simulink model "P4_Like"  (R2015b)
settings: Solver=VariableStepAuto  StartTime=0.0  StopTime=100  RelTol=1e-3
values from neighbouring files (symbols this model uses):
  B = 0.1    [Parameters.m]    (also in controller2.m = b/tsampling * eye(3,3))
  Dm = 0.2    [Parameters.m]
  Ds = 0.1    [Parameters.m]
  K = ceil(max(K1,K2))    [Gains.m]
  Lm1 = 0.5    [Parameters.m]
  Lm2 = 0.5    [Parameters.m]
  Ls1 = 0.5    [Parameters.m]
  Ls2 = 0.5    [Parameters.m]
  Mm1 = 1    [Parameters.m]
  Mm2 = 1    [Parameters.m]
  Ms1 = 2    [Parameters.m]
  Ms2 = 2    [Parameters.m]
  P = 10    [Parameters.m]
  q0 = [0;0]    [Parameters.m]
  v0 = [0;0;0]    [Initiation.m]    (also in Parameters.m = [0;0])
settings Model: Creator=TOSHIBA  LastModifiedBy=TOSHIBA

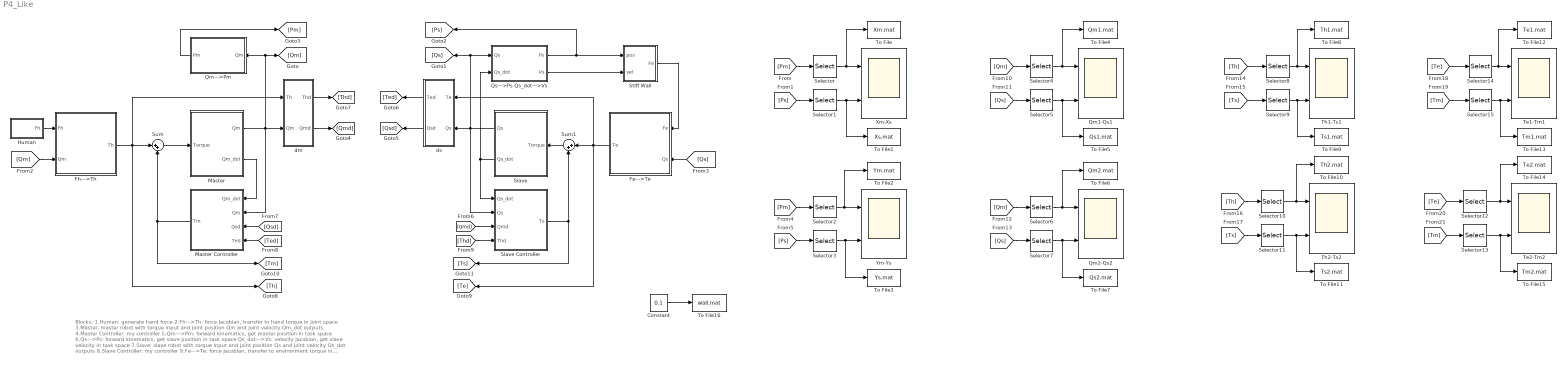
== system P4_Like ==
  note: Blocks:
      | 1.Human: generate hand force
      | 2.Fh--->Th: force Jacobian, transfer to hand torque in joint space
      | 3.Master: master robot with torque input and joint position Qm and joint velocity Qm_dot outputs
      | 4.Master Controller: my controller
      | 5.Qm--->Pm: forward kinematics, get master position in task space
      | 6.Qs--->Ps: forward kinematics, get slave position in task space
      | Qs_dot--->Vs: velocity jacobian, get slave velocity in task space
      | 7.Slave: slave robot with torque input and joint position Qs and joint velocity Qs_dot outputs
      | 8.Slave Controller: my controller
      | 9.Fe--->Te: force Jacobian, transfer to environment torque in joint space
      | 10.Stiff Wall: spring with k=10KN/m, active damping d=40Ns/m
  Constant : Constant  Value=0.1
  Fe--->Te : Subsystem
  Fh--->Th : Subsystem
  Human : Subsystem
  Master : Subsystem
  Master Controller : Subsystem
  Qm--->Pm : Subsystem
  Qm1-Qs1 : Scope  NumInputPorts=2
  Qm2-Qs2 : Scope  NumInputPorts=2
  Qs--->Ps Qs_dot--->Vs : Subsystem
  Selector{,1,4..5,8..9,14..15} (8 alike) : Selector  InputPortWidth=2  IndexOptions=Index vector (dialog)  Indices=[1]  OutputSizes=1
  Selector{2..3,6..7,10..13} (8 alike) : Selector  InputPortWidth=2  IndexOptions=Index vector (dialog)  Indices=[2]  OutputSizes=1
  Slave : Subsystem
  Slave Controller : Subsystem
  Stiff Wall : Subsystem
  Sum : Sum  Inputs=|++
  Sum1 : Sum  Inputs=|++
  Te1-Tm1 : Scope  NumInputPorts=2
  Te2-Tm2 : Scope  NumInputPorts=2
  Th1-Ts1 : Scope  NumInputPorts=2
  Th2-Ts2 : Scope  NumInputPorts=2
  To File : ToFile  Filename=Xm.mat  MatrixName=Xm  SaveFormat=Timeseries
  To File1 : ToFile  Filename=Xs.mat  MatrixName=Xs  SaveFormat=Timeseries
  To File10 : ToFile  Filename=Th2.mat  MatrixName=Th2  SaveFormat=Timeseries
  To File11 : ToFile  Filename=Ts2.mat  MatrixName=Ts2  SaveFormat=Timeseries
  To File12 : ToFile  Filename=Te1.mat  MatrixName=Te1  SaveFormat=Timeseries
  To File13 : ToFile  Filename=Tm1.mat  MatrixName=Tm1  SaveFormat=Timeseries
  To File14 : ToFile  Filename=Te2.mat  MatrixName=Te2  SaveFormat=Timeseries
  To File15 : ToFile  Filename=Tm2.mat  MatrixName=Tm2  SaveFormat=Timeseries
  To File16 : ToFile  Filename=wall.mat  MatrixName=wall  SaveFormat=Timeseries
  To File2 : ToFile  Filename=Ym.mat  MatrixName=Ym  SaveFormat=Timeseries
  To File3 : ToFile  Filename=Ys.mat  MatrixName=Ys  SaveFormat=Timeseries
  To File4 : ToFile  Filename=Qm1.mat  MatrixName=Qm1  SaveFormat=Timeseries
  To File5 : ToFile  Filename=Qs1.mat  MatrixName=Qs1  SaveFormat=Timeseries
  To File6 : ToFile  Filename=Qm2.mat  MatrixName=Qm2  SaveFormat=Timeseries
  To File7 : ToFile  Filename=Qs2.mat  MatrixName=Qs2  SaveFormat=Timeseries
  To File8 : ToFile  Filename=Th1.mat  MatrixName=Th1  SaveFormat=Timeseries
  To File9 : ToFile  Filename=Ts1.mat  MatrixName=Ts1  SaveFormat=Timeseries
  Xm-Xs : Scope  NumInputPorts=2
  Ym-Ys : Scope  NumInputPorts=2
  dm : Subsystem
  ds : Subsystem
  wires:
  Qs--->Ps Qs_dot--->Vs/1(Ps) -> Stiff Wall/1(pos), [Ps]
  Fe--->Te/1(Te) -> [Te], ds/1(Te), Sum1/1
  Sum1/1 -> Slave/1(Torque)
  Sum/1 -> Master/1(Torque)
  Fh--->Th/1(Th) -> [Th], dm/1(Th), Sum/1
  Master/2(Qm_dot) -> Master Controller/1(Qm_dot)
  Master Controller/1(Tm) -> [Tm], Sum/2
  Slave/2(Qs_dot) -> Qs--->Ps Qs_dot--->Vs/2(Qs_dot), Slave Controller/1(Qs_dot)
  Slave Controller/1(Ts) -> [Ts], Sum1/2
  [Qs] -> Fe--->Te/2(Qs)
  Master/1(Qm) -> Master Controller/2(Qm), dm/2(Qm), [Qm], Qm--->Pm/1(Qm)
  Slave/1(Qs) -> ds/2(Qs), [Qs], Qs--->Ps Qs_dot--->Vs/1(Qs), Slave Controller/2(Qs)
  [Qm] -> Fh--->Th/2(Qm)
  Human/1(Fh) -> Fh--->Th/1(Fh)
  Qm--->Pm/1(Pm) -> [Pm]
  [Pm] -> Selector/1
  Selector/1 -> To File/1, Xm-Xs/1
  [Ps] -> Selector1/1
  Selector1/1 -> To File1/1, Xm-Xs/2
  [Pm] -> Selector2/1
  Selector2/1 -> To File2/1, Ym-Ys/1
  [Ps] -> Selector3/1
  Selector3/1 -> To File3/1, Ym-Ys/2
  [Qmd] -> Slave Controller/3(Qmd)
  [Qsd] -> Master Controller/3(Qsd)
  [Ted] -> Master Controller/4(Ted)
  ds/2(Qsd) -> [Qsd]
  ds/1(Ted) -> [Ted]
  dm/2(Qmd) -> [Qmd]
  dm/1(Thd) -> [Thd]
  [Thd] -> Slave Controller/4(Thd)
  [Qs] -> Selector5/1
  [Qm] -> Selector4/1
  Selector4/1 -> To File4/1, Qm1-Qs1/1
  Selector5/1 -> To File5/1, Qm1-Qs1/2
  [Qs] -> Selector7/1
  [Qm] -> Selector6/1
  Selector6/1 -> To File6/1, Qm2-Qs2/1
  Selector7/1 -> To File7/1, Qm2-Qs2/2
  [Th] -> Selector8/1
  [Ts] -> Selector9/1
  Selector9/1 -> To File9/1, Th1-Ts1/2
  Selector8/1 -> To File8/1, Th1-Ts1/1
  [Ts] -> Selector11/1
  [Th] -> Selector10/1
  Selector10/1 -> To File10/1, Th2-Ts2/1
  [Te] -> Selector14/1
  [Tm] -> Selector15/1
  Selector15/1 -> To File13/1, Te1-Tm1/2
  Selector14/1 -> To File12/1, Te1-Tm1/1
  [Tm] -> Selector13/1
  [Te] -> Selector12/1
  Selector12/1 -> To File14/1, Te2-Tm2/1
  Selector13/1 -> To File15/1, Te2-Tm2/2
  Selector11/1 -> To File11/1, Th2-Ts2/2
  Constant/1 -> To File16/1
  Qs--->Ps Qs_dot--->Vs/2(Vs) -> Stiff Wall/2(vel)
  Stiff Wall/1(Fe) -> Fe--->Te/1(Fe)

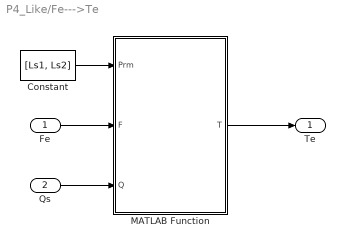
== system P4_Like/Fe--->Te ==
  Fe : Inport
  Qs : Inport  Port=2
  Constant : Constant  Value=[Ls1, Ls2]
  MATLAB Function : MATLAB Function  TreatAsAtomicUnit=on
  Te : Outport
  wires:
  Qs/1 -> MATLAB Function/3(Q)
  Fe/1 -> MATLAB Function/2(F)
  MATLAB Function/1(T) -> Te/1
  Constant/1 -> MATLAB Function/1(Prm)

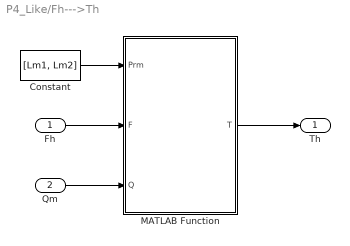
== system P4_Like/Fh--->Th ==
  Fh : Inport
  Qm : Inport  Port=2
  Constant : Constant  Value=[Lm1, Lm2]
  MATLAB Function : MATLAB Function  TreatAsAtomicUnit=on
  Th : Outport
  wires:
  Fh/1 -> MATLAB Function/2(F)
  MATLAB Function/1(T) -> Th/1
  Qm/1 -> MATLAB Function/3(Q)
  Constant/1 -> MATLAB Function/1(Prm)

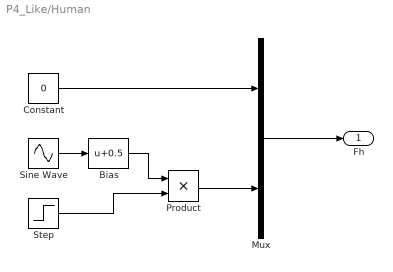
== system P4_Like/Human ==
  Bias : Bias  Bias=0.5
  Constant : Constant  Value=0
  Mux : Mux  Inputs=2
  Product : Product
  Sine Wave : Sin  Frequency=pi/20  SampleTime=0
  Step : Step  Time=100  Before=1  After=0  SampleTime=0
  Fh : Outport
  wires:
  Mux/1 -> Fh/1
  Constant/1 -> Mux/1
  Step/1 -> Product/2
  Bias/1 -> Product/1
  Product/1 -> Mux/2
  Sine Wave/1 -> Bias/1

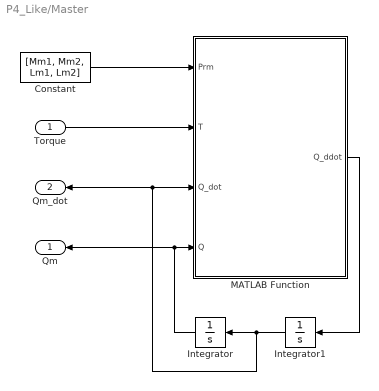
== system P4_Like/Master ==
  Torque : Inport
  Constant : Constant  Value=[Mm1, Mm2, Lm1, Lm2]
  Integrator : Integrator  InitialCondition=q0
  Integrator1 : Integrator  InitialCondition=v0
  MATLAB Function : MATLAB Function  TreatAsAtomicUnit=on
  Qm : Outport
  Qm_dot : Outport  Port=2
  wires:
  Torque/1 -> MATLAB Function/2(T)
  Constant/1 -> MATLAB Function/1(Prm)
  MATLAB Function/1(Q_ddot) -> Integrator1/1
  Integrator1/1 -> MATLAB Function/3(Q_dot), Qm_dot/1, Integrator/1
  Integrator/1 -> MATLAB Function/4(Q), Qm/1

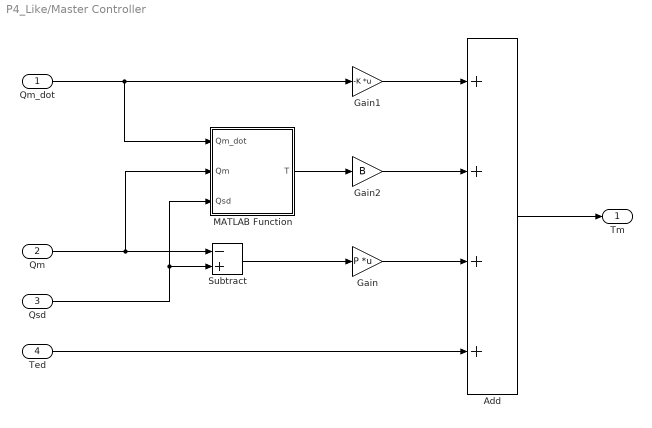
== system P4_Like/Master Controller ==
  Qm_dot : Inport
  Qm : Inport  Port=2
  Qsd : Inport  Port=3
  Ted : Inport  Port=4
  Add : Sum  Inputs=++++
  Gain : Gain  Gain=P  Multiplication=Matrix(K*u) (u vector)
  Gain1 : Gain  Gain=-K  Multiplication=Matrix(K*u) (u vector)
  Gain2 : Gain  Gain=B
  MATLAB Function : MATLAB Function  TreatAsAtomicUnit=on
  Subtract : Sum  Inputs=-+
  Tm : Outport
  wires:
  Qm/1 -> MATLAB Function/2(Qm), Subtract/1
  Qsd/1 -> Subtract/2, MATLAB Function/3(Qsd)
  Gain/1 -> Add/3
  Gain1/1 -> Add/1
  Add/1 -> Tm/1
  Qm_dot/1 -> MATLAB Function/1(Qm_dot), Gain1/1
  Subtract/1 -> Gain/1
  Ted/1 -> Add/4
  MATLAB Function/1(T) -> Gain2/1
  Gain2/1 -> Add/2

== system P4_Like/Qm--->Pm ==
  Qm : Inport
  MATLAB Function : MATLAB Function  TreatAsAtomicUnit=on
  Prm : Constant  Value=[Lm1, Lm2]
  Pm : Outport
  wires:
  MATLAB Function/1(Pos) -> Pm/1
  Qm/1 -> MATLAB Function/2(Q)
  Prm/1 -> MATLAB Function/1(Prm)

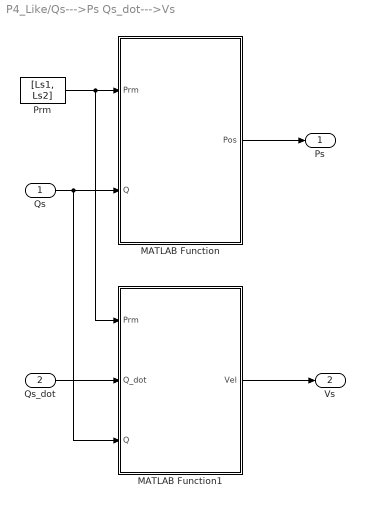
== system P4_Like/Qs--->Ps Qs_dot--->Vs ==
  Qs : Inport
  Qs_dot : Inport  Port=2
  MATLAB Function : MATLAB Function  TreatAsAtomicUnit=on
  MATLAB Function1 : MATLAB Function  TreatAsAtomicUnit=on
  Prm : Constant  Value=[Ls1, Ls2]
  Ps : Outport
  Vs : Outport  Port=2
  wires:
  Qs/1 -> MATLAB Function1/3(Q), MATLAB Function/2(Q)
  MATLAB Function/1(Pos) -> Ps/1
  Prm/1 -> MATLAB Function1/1(Prm), MATLAB Function/1(Prm)
  Qs_dot/1 -> MATLAB Function1/2(Q_dot)
  MATLAB Function1/1(Vel) -> Vs/1

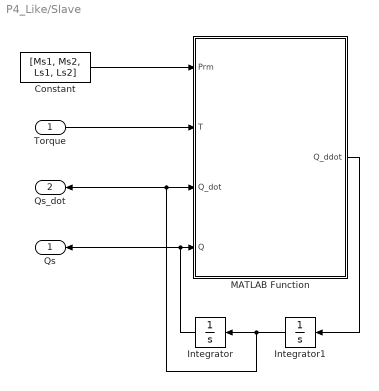
== system P4_Like/Slave ==
  Torque : Inport
  Constant : Constant  Value=[Ms1, Ms2, Ls1, Ls2]
  Integrator : Integrator  InitialCondition=q0
  Integrator1 : Integrator  InitialCondition=v0
  MATLAB Function : MATLAB Function  TreatAsAtomicUnit=on
  Qs : Outport
  Qs_dot : Outport  Port=2
  wires:
  Torque/1 -> MATLAB Function/2(T)
  Constant/1 -> MATLAB Function/1(Prm)
  MATLAB Function/1(Q_ddot) -> Integrator1/1
  Integrator1/1 -> Qs_dot/1, MATLAB Function/3(Q_dot), Integrator/1
  Integrator/1 -> Qs/1, MATLAB Function/4(Q)

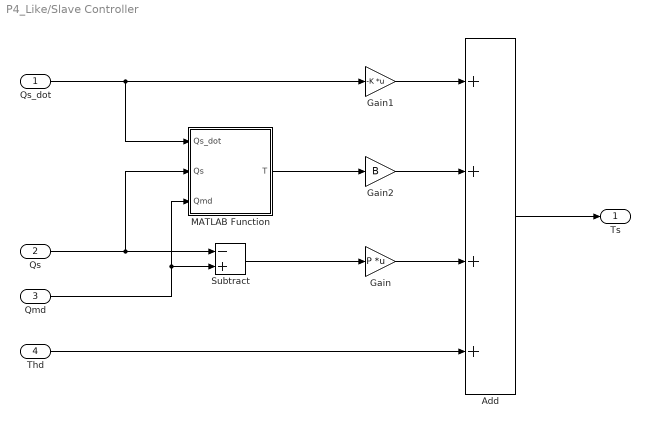
== system P4_Like/Slave Controller ==
  Qs_dot : Inport
  Qs : Inport  Port=2
  Qmd : Inport  Port=3
  Thd : Inport  Port=4
  Add : Sum  Inputs=++++
  Gain : Gain  Gain=P  Multiplication=Matrix(K*u) (u vector)
  Gain1 : Gain  Gain=-K  Multiplication=Matrix(K*u) (u vector)
  Gain2 : Gain  Gain=B
  MATLAB Function : MATLAB Function  TreatAsAtomicUnit=on
  Subtract : Sum  Inputs=-+
  Ts : Outport
  wires:
  Subtract/1 -> Gain/1
  Qs_dot/1 -> MATLAB Function/1(Qs_dot), Gain1/1
  Add/1 -> Ts/1
  Gain1/1 -> Add/1
  Qmd/1 -> MATLAB Function/3(Qmd), Subtract/2
  Qs/1 -> MATLAB Function/2(Qs), Subtract/1
  Gain/1 -> Add/3
  Thd/1 -> Add/4
  Gain2/1 -> Add/2
  MATLAB Function/1(T) -> Gain2/1

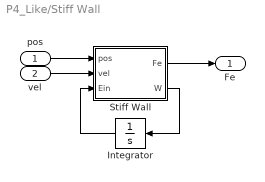
== system P4_Like/Stiff Wall ==
  pos : Inport
  vel : Inport  Port=2
  Integrator : Integrator
  Stiff Wall : MATLAB Function  TreatAsAtomicUnit=on
  Fe : Outport
  wires:
  Stiff Wall/1(Fe) -> Fe/1
  Stiff Wall/2(W) -> Integrator/1
  Integrator/1 -> Stiff Wall/3(Ein)
  vel/1 -> Stiff Wall/2(vel)
  pos/1 -> Stiff Wall/1(pos)

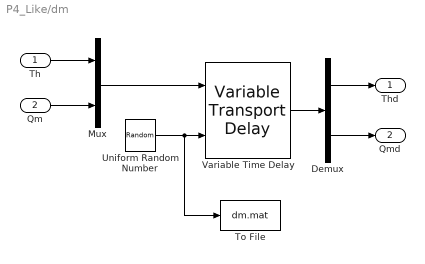
== system P4_Like/dm ==
  Th : Inport
  Qm : Inport  Port=2
  Demux : Demux  Outputs=2
  Mux : Mux  Inputs=2
  To File : ToFile  Filename=dm.mat  MatrixName=dm  SaveFormat=Timeseries
  Uniform Random Number : UniformRandomNumber  Minimum=0  Maximum=Dm  SampleTime=0.1
  Variable Time Delay : VariableTransportDelay  MaximumDelay=Dm
  Thd : Outport
  Qmd : Outport  Port=2
  wires:
  Uniform Random Number/1 -> Variable Time Delay/2, To File/1
  Mux/1 -> Variable Time Delay/1
  Th/1 -> Mux/1
  Qm/1 -> Mux/2
  Variable Time Delay/1 -> Demux/1
  Demux/1 -> Thd/1
  Demux/2 -> Qmd/1

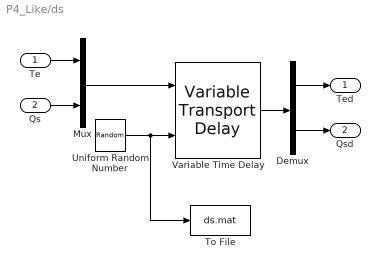
== system P4_Like/ds ==
  Te : Inport
  Qs : Inport  Port=2
  Demux : Demux  Outputs=2
  Mux : Mux  Inputs=2
  To File : ToFile  Filename=ds.mat  MatrixName=ds  SaveFormat=Timeseries
  Uniform Random Number : UniformRandomNumber  Minimum=0  Maximum=Ds  SampleTime=0.1
  Variable Time Delay : VariableTransportDelay  MaximumDelay=Ds
  Ted : Outport
  Qsd : Outport  Port=2
  wires:
  Uniform Random Number/1 -> To File/1, Variable Time Delay/2
  Mux/1 -> Variable Time Delay/1
  Variable Time Delay/1 -> Demux/1
  Te/1 -> Mux/1
  Qs/1 -> Mux/2
  Demux/1 -> Ted/1
  Demux/2 -> Qsd/1

== matlab function P4_Like/Master/MATLAB Function ==
  data: Prm input; Q_ddot output; T input; Q_dot input; Q input
function Q_ddot  = RobotArm_2DOF(Prm, T, Q_dot, Q)
%#codegen
g = 9.8;
m1 = Prm(1);
m2 = Prm(2);
l1 = Prm(3);
l2 = Prm(4);
q1 = Q(1);
q2 = Q(2);
q1_dot = Q_dot(1);
q2_dot = Q_dot(2);
M11 = m2*l2^2+(m1+m2)*l1^2+2*m2*l1*l2*cos(q2);
M12 = m2*l2^2+m2*l1*l2*cos(q2);
M21 = M12;
M22 = m2*l2^2;
M = [M11, M12; M21, M22];
C11 = -2*m2*l1*l2*sin(q2)*q2_dot;
C12 = -m2*l1*l2*sin(q2)*q2_dot;
C21 = m2*l1*l2*sin(q2)*q1_dot;
C22 = 0;
C = [C11, C12; C21, C22];
g1 = m2*g*l2*sin(q1+q2)+(m1+m2)*g*l1*sin(q1);
g2 = m2*g*l2*sin(q1+q2);
G = [g1; g2];
Q_ddot = M\(T-C*Q_dot);

== matlab function P4_Like/Stiff Wall/Stiff Wall ==
  data: pos input; Fe output; vel input; Ein input; W output
function [Fe, W]  = Envir(pos,vel,Ein)
%#codegen
kWall = 10000;
bWall = 40;
if pos(2)>=0.1
    Fk=[0; -(pos(2)-0.1)*kWall];
    %Fb = zeros(2,1);
    if Ein<=0.5;
        Fb=bWall*[0;vel(2)];
    else
        Fb=zeros(2,1);
    end
    %}
    Fe=Fk+Fb;
    
    W=Fb'*vel;
else
    Fe=zeros(2,1);
    W=0;
end

== matlab function P4_Like/Slave/MATLAB Function ==
  data: Prm input; Q_ddot output; T input; Q_dot input; Q input
function Q_ddot  = RobotArm_2DOF(Prm, T, Q_dot, Q)
%#codegen
g = 9.8;
m1 = Prm(1);
m2 = Prm(2);
l1 = Prm(3);
l2 = Prm(4);
q1 = Q(1);
q2 = Q(2);
q1_dot = Q_dot(1);
q2_dot = Q_dot(2);
M11 = m2*l2^2+(m1+m2)*l1^2+2*m2*l1*l2*cos(q2);
M12 = m2*l2^2+m2*l1*l2*cos(q2);
M21 = M12;
M22 = m2*l2^2;
M = [M11, M12; M21, M22];
C11 = -2*m2*l1*l2*sin(q2)*q2_dot;
C12 = -m2*l1*l2*sin(q2)*q2_dot;
C21 = m2*l1*l2*sin(q2)*q1_dot;
C22 = 0;
C = [C11, C12; C21, C22];
g1 = m2*g*l2*sin(q1+q2)+(m1+m2)*g*l1*sin(q1);
g2 = m2*g*l2*sin(q1+q2);
G = [g1; g2];
Q_ddot = M\(T-C*Q_dot);

== matlab function P4_Like/Qm--->Pm/MATLAB Function ==
  data: Prm input; Pos output; Q input
function Pos = ForwardKinematics(Prm, Q)
%#codegen
l1 = Prm(1);
l2 = Prm(2);
q1 = Q(1);
q2 = Q(2);
x = l1*cos(q1)+l2*cos(q1+q2);
y = l1*sin(q1)+l2*sin(q1+q2);
Pos = [x; y];

== matlab function P4_Like/Qs--->Ps Qs_dot--->Vs/MATLAB Function ==
  data: Prm input; Pos output; Q input
function Pos = ForwardKinematics(Prm, Q)
%#codegen
l1 = Prm(1);
l2 = Prm(2);
q1 = Q(1);
q2 = Q(2);
x = l1*cos(q1)+l2*cos(q1+q2);
y = l1*sin(q1)+l2*sin(q1+q2);
Pos = [x; y];

== matlab function P4_Like/Fh--->Th/MATLAB Function ==
  data: Prm input; T output; F input; Q input
function T = Force_to_Torque(Prm, F, Q)
%#codegen
l1 = Prm(1);
l2 = Prm(2);
q1 = Q(1);
q2 = Q(2);
J11 = -l1*sin(q1)-l2*sin(q1+q2);
J12 = -l2*sin(q1+q2);
J21 = l1*cos(q1)+l2*cos(q1+q2);
J22 = l2*cos(q1+q2);
J = [J11, J12; J21, J22];
T = J'*F;

== matlab function P4_Like/Fe--->Te/MATLAB Function ==
  data: Prm input; T output; F input; Q input
function T = Force_to_Torque(Prm, F, Q)
%#codegen
l1 = Prm(1);
l2 = Prm(2);
q1 = Q(1);
q2 = Q(2);
J11 = -l1*sin(q1)-l2*sin(q1+q2);
J12 = -l2*sin(q1+q2);
J21 = l1*cos(q1)+l2*cos(q1+q2);
J22 = l2*cos(q1+q2);
J = [J11, J12; J21, J22];
T = J'*F;

== matlab function P4_Like/Slave Controller/MATLAB Function ==
  data: Qs_dot input; T output; Qs input; Qmd input
function T = fcn(Qs_dot, Qs, Qmd)
%#codegen
if Qs_dot(1)~=0 && Qs_dot(2)~=0
    T=-(0.5./Qs_dot)*((Qs-Qmd)'*(Qs-Qmd));
elseif Qs_dot(1)==0 &&Qs_dot(2)==0
    T=zeros(2,1);
elseif Qs_dot(1)~=0 && Qs_dot(2)==0
    T=-[1/Qs_dot(1);0]*((Qs-Qmd)'*(Qs-Qmd));
else
    T=-[0;1/Qs_dot(2)]*((Qs-Qmd)'*(Qs-Qmd));
end

== matlab function P4_Like/Master Controller/MATLAB Function ==
  data: Qm_dot input; T output; Qm input; Qsd input
function T = fcn(Qm_dot, Qm, Qsd)
%#codegen
if Qm_dot(1)~=0 && Qm_dot(2)~=0
    T=-(0.5./Qm_dot)*((Qm-Qsd)'*(Qm-Qsd));
elseif Qm_dot(1)==0 && Qm_dot(2)==0
    T=zeros(2,1);
elseif Qm_dot(1)~=0 && Qm_dot(2)==0
    T=-[1/Qm_dot(1);0]*((Qm-Qsd)'*(Qm-Qsd));
else
    T=-[0;1/Qm_dot(2)]*((Qm-Qsd)'*(Qm-Qsd));
end

== matlab function P4_Like/Qs--->Ps Qs_dot--->Vs/MATLAB Function1 ==
  data: Prm input; Vel output; Q_dot input; Q input
function Vel = Velocity_Jacobian(Prm, Q_dot, Q)
%#codegen
l1 = Prm(1);
l2 = Prm(2);
q1 = Q(1);
q2 = Q(2);
J11 = -l1*sin(q1)-l2*sin(q1+q2);
J12 = -l2*sin(q1+q2);
J21 = l1*cos(q1)+l2*cos(q1+q2);
J22 = l2*cos(q1+q2);
J = [J11, J12; J21, J22];
Vel=J*Q_dot;
